simulink model "robot_etu"  (R2017a)
settings: Solver=VariableStepAuto  StartTime=t0  StopTime=tf  RelTol=1e-3
undefined symbols (not defined in the file): K, ue, x0, xe
settings Model: Creator=lgirodon  LastModifiedBy=lgirodon

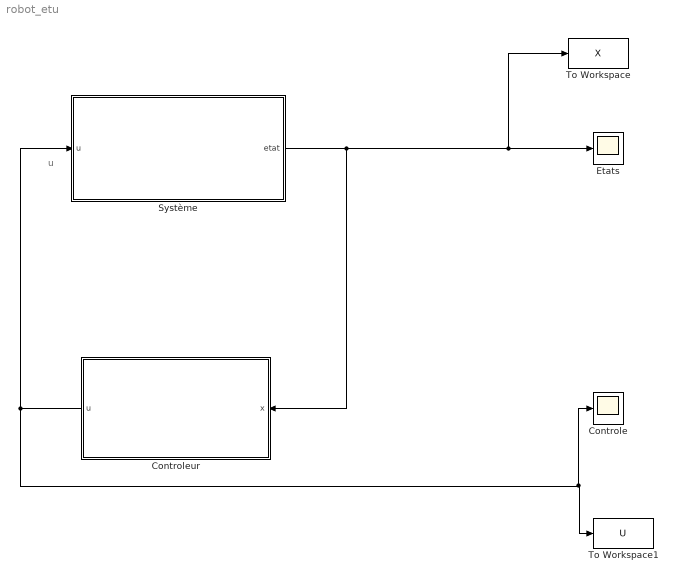
== system robot_etu ==
  note: u
  Controle : Scope
  Controleur : Subsystem
  Etats : Scope
  Système : Subsystem
  To Workspace : ToWorkspace  VariableName=X  SaveFormat=Timeseries  SampleTime=-1
  To Workspace1 : ToWorkspace  VariableName=U  SaveFormat=Timeseries  SampleTime=-1
  wires:
  Controleur/1(u) -> To Workspace1/1, Controle/1, Système/1(u)
  Système/1(etat) -> To Workspace/1, Etats/1, Controleur/1(x)

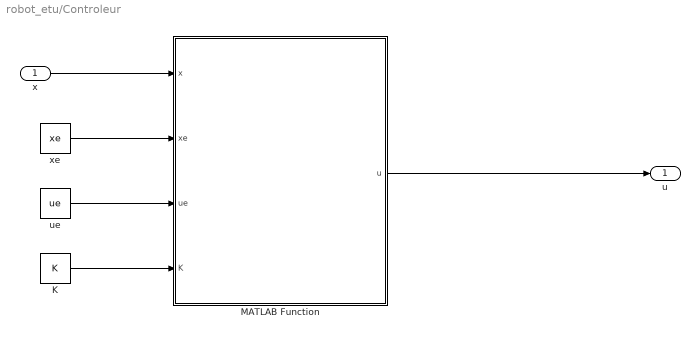
== system robot_etu/Controleur ==
  x : Inport
  K : Constant  Value=K
  MATLAB Function : MATLAB Function  TreatAsAtomicUnit=on
  ue : Constant  Value=ue
  xe : Constant  Value=xe
  u : Outport
  wires:
  x/1 -> MATLAB Function/1(x)
  xe/1 -> MATLAB Function/2(xe)
  ue/1 -> MATLAB Function/3(ue)
  K/1 -> MATLAB Function/4(K)
  MATLAB Function/1(u) -> u/1

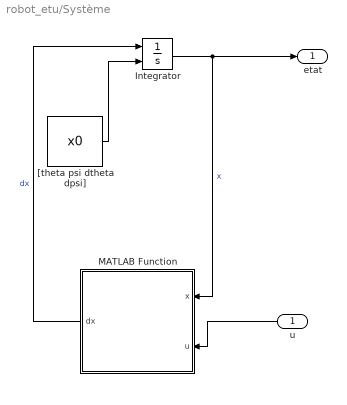
== system robot_etu/Système ==
  u : Inport
  Integrator : Integrator  InitialConditionSource=external
  MATLAB Function : MATLAB Function  TreatAsAtomicUnit=on
  "[theta psi dtheta dpsi]" : Constant  Value=x0
  etat : Outport
  wires:
  Integrator/1 -> etat/1, MATLAB Function/1(x)  "x"
  MATLAB Function/1(dx) -> Integrator/1  "dx"
  "[theta psi dtheta dpsi]"/1 -> Integrator/2
  u/1 -> MATLAB Function/2(u)

== matlab function robot_etu/Système/MATLAB Function ==
  data: x input; dx output; u input
function dx   = fonction( x, u)
%   Dynamic equations of motion of the segway on an axis.
%   Inputs: - x = [theta psi dtheta dpsi]
%               theta: average angle of the wheels      [rad]
%               psi: body pitch angle                   [rad]
%               dtheta: average velocity of the wheels  [rad/s]
%               dpsi: body pitch velocity               [rad/s]
%          - u: DC motor voltage (same value for both motors) [V]

    % State
    psi = x(2);
    dtheta = x(3);
    dpsi = x(4);

    % Parameters
    
    g = 9.81;           % gravity acceleration [m/sec^2]
    m = 0.03;           % wheel weight [kg]
    R = 0.04;           % wheel radius [m]
    Jw = m*R^2/2;       % wheel inertia moment [kg*m^2]
    M = 0.6;            % body weight [kg]
    H = 0.144;          % body height [m]
    L = H/2;            % distance of the center of mass from the wheel axle [m]
    Jpsi = M*L^2/3;     % body pitch inertia [kgm^2]
    Jm = 1e-5;          % DC motor inertia moment [kgm^2]
    Rm = 6.69;          % DC motor resistance [Ohm]
    Kb = 0.468;         % DC motor back EMF constant [Vsec/rad]
    Kt = 0.317;         % DC motor torque constant [Nm/A]
    n = 1;              % gear ratio
    fm = 0.0022;        % friction coefficient between body and DC motor
    fw = 0;             % friction coefficient between wheel and floor
    
    % Equations of motion
    c1 = (2*m+M)*R^2 + 2*Jw + 2*n^2*Jm;
    c2 = M*L*R*cos(psi) - 2*n^2*Jm;
    c3 = -M*L*R*dpsi^2*sin(psi);
    c4 = M*L^2 + Jpsi + 2*n^2*Jm;
    c5 = -M*g*L*sin(psi);

    alpha = Kt/Rm;
    beta = Kt*Kb/Rm + fm;

    Ftheta = alpha*(2*u) - 2*(beta+fw)*dtheta + 2*beta*dpsi;
    Fpsi = -alpha*(2*u) + 2*beta*dtheta - 2*beta*dpsi;

    ddtheta = (c4*c3 - c2*c5 + c4*Ftheta - c2*Fpsi)/(c4*c1 - c2^2);
    ddpsi = (Fpsi- c2*ddtheta - c5)/c4;
    dx = [dtheta dpsi ddtheta ddpsi]';

end

== matlab function robot_etu/Controleur/MATLAB Function ==
  data: x input; u output; xe input; ue input; K input
function u = fcn(x,xe,ue,K)
u=ue+(K(:)')*(x(:)-xe(:));
end
